simulink model "Exercitiul_2_Simulink"  (R2021b)
settings: Solver=VariableStepAuto  StartTime=0.0  StopTime=10.0  RelTol=1e-3

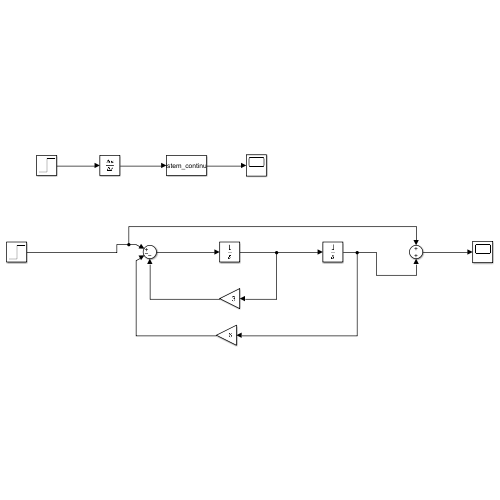
[thumbnail: Simulink's stored preview of the top-level diagram]
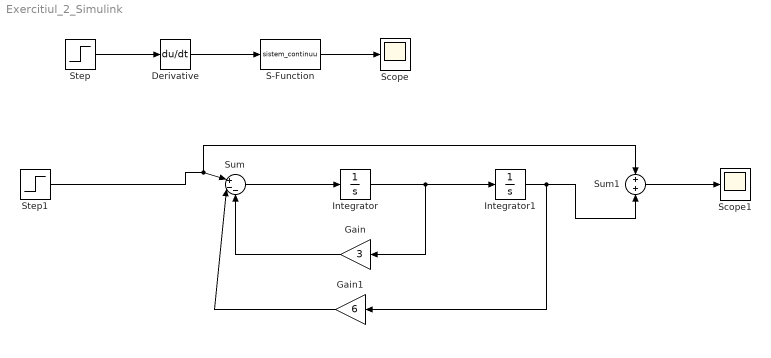
== system Exercitiul_2_Simulink ==
  Derivative : Derivative
  Gain : Gain  Gain=3
  Gain1 : Gain  Gain=6
  Integrator : Integrator
  Integrator1 : Integrator
  S-Function : S-Function  FunctionName=sistem_continuu  Parameters=A, B, C  SFunctionDeploymentMode=off  EnableBusSupport=off
  Scope : Scope
  Scope1 : Scope
  Step : Step  SampleTime=0
  Step1 : Step  SampleTime=0
  Sum : Sum  Inputs=|+--
  Sum1 : Sum  Inputs=+|+
  wires:
  Step/1 -> Derivative/1
  Derivative/1 -> S-Function/1
  S-Function/1 -> Scope/1
  Step1/1 -> Sum1/1, Sum/1
  Sum/1 -> Integrator/1
  Integrator/1 -> Gain/1, Integrator1/1
  Integrator1/1 -> Gain1/1, Sum1/2
  Gain/1 -> Sum/3
  Gain1/1 -> Sum/2
  Sum1/1 -> Scope1/1
